simulink model "speed_control"  (R2024b)
settings: Solver=VariableStepAuto  StartTime=0.0  StopTime=10.0  RelTol=1e-3
values from neighbouring files (symbols this model uses):
  pmsm =     [foc.mat]    (also in inverter.mat; speed_control.mat; vbyf.mat)
  Ts = 2.5e-05    [foc.mat]    (also in inverter.mat; speed_control.mat; vbyf.mat)
libraries: mcbcontrollergainlib x2, mcbfoclib x1, mcbpositiondecoderlib x1, mcbplantlib x1, autolibpmsminterior x1, slpidlib x1
settings Model: Creator=realf  LastModifiedBy=realf

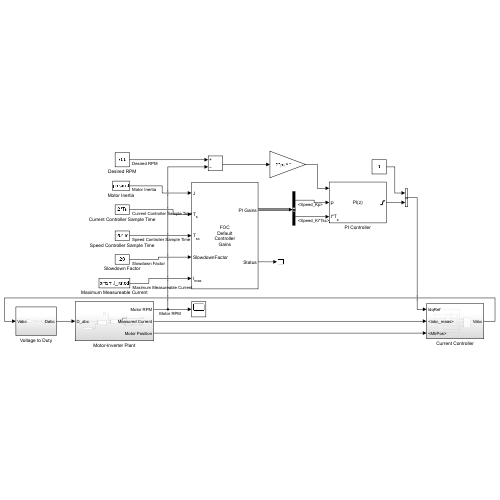
[thumbnail: Simulink's stored preview of the top-level diagram]
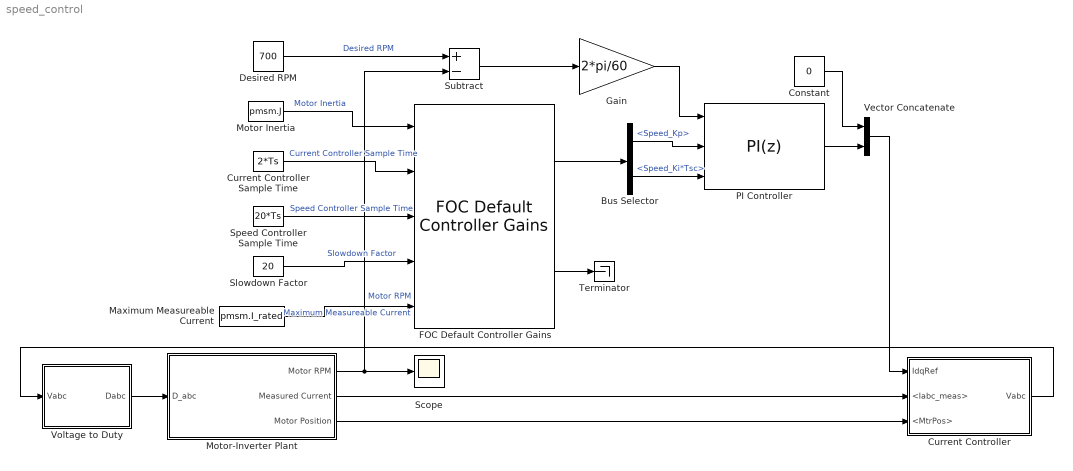
== system speed_control ==
  Bus Selector : BusSelector  OutputSignals=Speed_Kp,Speed_Ki*Tsc
  Constant : Constant  Value=0
  Current Controller : Subsystem
  Current Controller Sample Time : Constant  Value=2*Ts
  Desired RPM : Constant  Value=700
  FOC Default Controller Gains : mcbcontrollergainlib/FOC Default Controller Gains  motorSelection=PMSM  unitType=SI Unit  outCurrentControlGain=off  outFWCGain=off  outSpeedControlGain=on  externalDelay=off  currentSensorDelay=50e-6  speedSensorDelay=50e-6  speedFilterDelay=0.02
      settings: LibrarySourceBlock=mcblib/Controls/Controllers/FOC Default Controller Gains
  Gain : Gain  Gain=2*pi/60
  Maximum Measureable Current : Constant  Value=pmsm.I_rated
  Motor Inertia : Constant  Value=pmsm.J
  Motor-Inverter Plant : Subsystem
  PI Controller : slpidlib/PID Controller  Controller=PI  Form=Parallel  TimeDomain=Discrete-time  UseExternalTs=off  SampleTime=-1  IntegratorMethod=Forward Euler  FilterMethod=Forward Euler  ControllerParametersSource=external  P=1  I=1  UseKiTs=on  D=0  UseExternalDerivativeSource=off  N=100  UseFilter=on  TunerSelectOption=Transfer Function Based (PID Tuner App)  InitialConditionSource=internal  InitialConditionForIntegrator=0  InitialConditionForFilter=0  DifferentiatorICPrevScaledInput=0  ExternalReset=none  TrackingMode=off  Kt=1  LimitOutput=on  SatLimitsSource=internal  UpperSaturationLimit=pmsm.I_rated  LowerSaturationLimit=-pmsm.I_rated  LinearizeAsGain=on  AntiWindupMode=clamping  Kb=1  LimitIntegrator=on  UpperIntegratorSaturationLimit=pmsm.I_rated  LowerIntegratorSaturationLimit=-pmsm.I_rated  RndMeth=Simplest  POutMin=[]  POutMax=[]  IOutMin=[]  IOutMax=[]  DOutMin=[]  DOutMax=[]  NOutMin=[]  NOutMax=[]  SumOutMin=[]  SumOutMax=[]  SaturationOutDataTypeStr=Inherit: Inherit via back propagation  SaturationOutMin=[]  SaturationOutMax=[]  PParamMin=[]  PParamMax=[]  IParamMin=[]  IParamMax=[]  DParamMin=[]  DParamMax=[]  NParamMin=[]  NParamMax=[]  KbParamMin=[]  KbParamMax=[]  KtParamMin=[]  KtParamMax=[]  KbOutMin=[]  KbOutMax=[]  KtOutMin=[]  KtOutMax=[]  IntegratorOutMin=[]  IntegratorOutMax=[]  FilterOutMin=[]  FilterOutMax=[]  SumI1OutMin=[]  SumI1OutMax=[]  SumI2OutMin=[]  SumI2OutMax=[]  SumI3OutMin=[]  SumI3OutMax=[]  SumI4OutMin=[]  SumI4OutMax=[]  SumDOutMin=[]  SumDOutMax=[]  DifferentiatorOutMin=[]  DifferentiatorOutMax=[]  FilterDiffOutCoefMin=[]  FilterDiffOutCoefMax=[]  ReciprocalOutMin=[]  ReciprocalOutMax=[]  SumDenOutMin=[]  SumDenOutMax=[]  SumNumOutMin=[]  SumNumOutMax=[]  DivideOutMin=[]  DivideOutMax=[]  UdiffTsProdOutMin=[]  UdiffTsProdOutMax=[]  NTsProdOutMin=[]  NTsProdOutMax=[]  UintegralTsProdOutMin=[]  UintegralTsProdOutMax=[]  UngainTsProdOutMin=[]  UngainTsProdOutMax=[]  ClampingZeroOutDataTypeStr=Inherit: Inherit via back propagation  ClampingZeroOutMin=[]  ClampingZeroOutMax=[]  FilterDenConstantOutDataTypeStr=Inherit: Inherit via back propagation  FilterDenConstantOutMin=[]  FilterDenConstantOutMax=[]  PCopyOutDataTypeStr=Inherit: Inherit via back propagation  PCopyOutMin=[]  PCopyOutMax=[]  NCopyOutDataTypeStr=Inherit: Inherit via back propagation  NCopyOutMin=[]  NCopyOutMax=[]  IntegratorContinuousStateAttributes=''  IntegratorStateMustResolveToSignalObject=off  IntegratorRTWStateStorageClass=Auto  FilterContinuousStateAttributes=''  FilterStateMustResolveToSignalObject=off  FilterRTWStateStorageClass=Auto  ParallelPVariant=ExternalParameters  IdealPVariant=Disabled  IVariant=ExternalParameters  DVariant=Disabled  IntegratorVariant=Discrete  SatVariant=Enabled  AWVariant=DiscClampingParallel  PCopyVariant=Disabled  TRVariant=Disabled  FdbkBlocksVariant=Forward  IdealPFdbkVariant=Disabled  SatFdbkVariant=Disabled  DerivativeFilterVariant=Disabled  NVariant=Disabled  NCopyVariant=Disabled_SignalSpec  FilterICVariant=Disabled  IntegratorICVariant=InternalICs  ExternalResetVariant=Disabled  TRSumVariant=Passthrough  SumFdbkVariant=Disabled  SumVariant=Sum_PI  TsampFilterVariant=InternalTs  TsampNgainVariant=Passthrough  TsampIntegralVariant=Disabled_SignalSpec  ExternalSaturationOutDataTypeStr=Inherit: Same as second input  DerivativeSourceVariant=Disabled  PreIntVariant=InternalPreInt
      settings: LibrarySourceBlock=mcbhdllib/Controls/Controllers/PI Controller
  Scope : Scope
  Slowdown Factor : Constant  Value=20
  Speed Controller Sample Time : Constant  Value=20*Ts
  Subtract : Sum  Inputs=+-
  Terminator : Terminator
  Vector Concatenate : Concatenate
  Voltage to Duty : Subsystem
  wires:
  Voltage to Duty/1(Dabc) -> Motor-Inverter Plant/1(D_abc)
  Current Controller Sample Time/1 -> FOC Default Controller Gains/2  "Current Controller Sample Time"
  Constant/1 -> Vector Concatenate/1
  Desired RPM/1 -> Subtract/1  "Desired RPM"
  Motor-Inverter Plant/1(Motor RPM) -> Scope/1, Subtract/2  "Motor RPM"
  Maximum Measureable Current/1 -> FOC Default Controller Gains/5  "Maximum Measureable Current"
  Motor-Inverter Plant/2(Measured Current) -> Current Controller/2(<Iabc_meas>)
  Motor Inertia/1 -> FOC Default Controller Gains/1  "Motor Inertia"
  Slowdown Factor/1 -> FOC Default Controller Gains/4  "Slowdown Factor"
  PI Controller/1 -> Vector Concatenate/2
  Speed Controller Sample Time/1 -> FOC Default Controller Gains/3  "Speed Controller Sample Time"
  Motor-Inverter Plant/3(Motor Position) -> Current Controller/3(<MtrPos>)
  Subtract/1 -> Gain/1
  FOC Default Controller Gains/1 -> Bus Selector/1
  FOC Default Controller Gains/2 -> Terminator/1
  Gain/1 -> PI Controller/1
  Bus Selector/1 -> PI Controller/2  "<Speed_Kp>"
  Bus Selector/2 -> PI Controller/3  "<Speed_Ki*Tsc>"
  Vector Concatenate/1 -> Current Controller/1(IdqRef)
  Current Controller/1(Vabc) -> Voltage to Duty/1(Vabc)

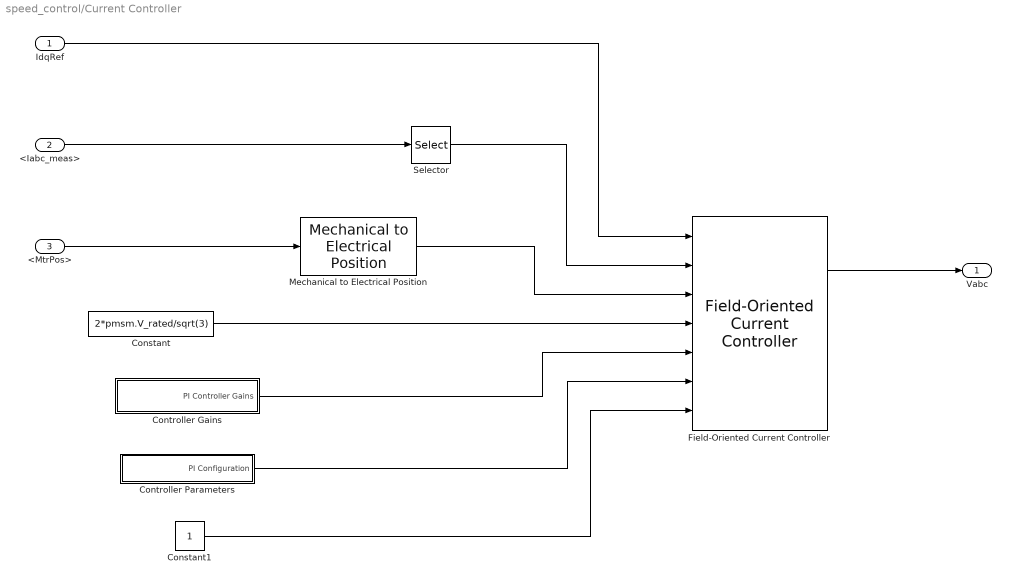
== system speed_control/Current Controller ==
  IdqRef : Inport
  <Iabc_meas> : Inport  Port=2
  <MtrPos> : Inport  Port=3
  Constant : Constant  Value=2*pmsm.V_rated/sqrt(3)
  Constant1 : Constant
  Controller Gains : Subsystem
  Controller Parameters : Subsystem
  Field-Oriented Current Controller : mcbfoclib/Field-Oriented Current Controller  AngleUnit=Radians  NumberOfLUTPoints=1024  AxisAlignment=D-axis  SaturationMethod=D-Q equivalence  PWMMethod=SVM: space vector modulation
  Mechanical to Electrical Position : mcbpositiondecoderlib/Mechanical to Electrical Position  PolePairsInputType=Specify via dialog  NrPP=pmsm.p  selectedRange=Radians  MechOfstInputType=Specify via dialog  mechOffsetIn=0  maxAngleIn=2*pi  InputDataType=single  VariantSelect=floating-point
  Selector : Selector  InputPortWidth=3  IndexOptions=Index vector (dialog)  Indices=[1 2]  OutputSizes=1
  Vabc : Outport
  wires:
  Field-Oriented Current Controller/1 -> Vabc/1
  <MtrPos>/1 -> Mechanical to Electrical Position/1
  IdqRef/1 -> Field-Oriented Current Controller/1
  <Iabc_meas>/1 -> Selector/1
  Controller Parameters/1(PI Configuration) -> Field-Oriented Current Controller/6
  Constant1/1 -> Field-Oriented Current Controller/7
  Selector/1 -> Field-Oriented Current Controller/2
  Constant/1 -> Field-Oriented Current Controller/4
  Controller Gains/1(PI Controller Gains) -> Field-Oriented Current Controller/5
  Mechanical to Electrical Position/1 -> Field-Oriented Current Controller/3

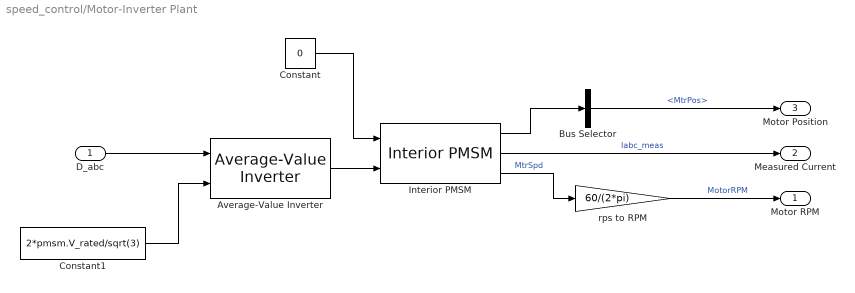
== system speed_control/Motor-Inverter Plant ==
  D_abc : Inport
  Average-Value Inverter : mcbplantlib/Average-Value Inverter
  Bus Selector : BusSelector  OutputSignals=MtrPos
  Constant : Constant  Value=0
  Constant1 : Constant  Value=2*pmsm.V_rated/sqrt(3)
  Interior PMSM : autolibpmsminterior/Interior PMSM  port_config=Torque  sim_type=Discrete  Ts=Ts  P=pmsm.p  Rs=pmsm.Rs  Ldq=[pmsm.Ld, pmsm.Lq]  KConstText=Permanent flux linkage constant (lambda_pm):  lambda_pm=pmsm.FluxPM  Ke=159.9771  mechanical=[pmsm.J, 0, 0]  idq0=[0 0]  theta_init=0  omega_init=0  KConst=pmsm.FluxPM  lambda_pm_calc=pmsm.FluxPM  Kt=0.07  RefBlkName='autolibpmsminterior/Interior PMSM'  aMode=5
  rps to RPM : Gain  Gain=60/(2*pi)
  Motor RPM : Outport
  Measured Current : Outport  Port=2
  Motor Position : Outport  Port=3
  wires:
  D_abc/1 -> Average-Value Inverter/1
  Interior PMSM/2 -> Measured Current/1  "Iabc_meas"
  Bus Selector/1 -> Motor Position/1  "<MtrPos>"
  Interior PMSM/1 -> Bus Selector/1
  Constant/1 -> Interior PMSM/1
  Constant1/1 -> Average-Value Inverter/2
  Average-Value Inverter/1 -> Interior PMSM/2
  rps to RPM/1 -> Motor RPM/1  "MotorRPM"
  Interior PMSM/3 -> rps to RPM/1  "MtrSpd"

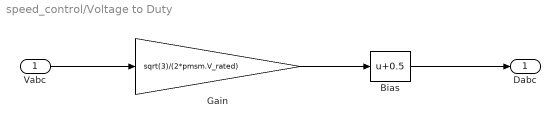
== system speed_control/Voltage to Duty ==
  Vabc : Inport
  Bias : Bias  Bias=0.5  SaturateOnIntegerOverflow=off
  Gain : Gain  Gain=sqrt(3)/(2*pmsm.V_rated)
  Dabc : Outport
  wires:
  Gain/1 -> Bias/1
  Vabc/1 -> Gain/1
  Bias/1 -> Dabc/1

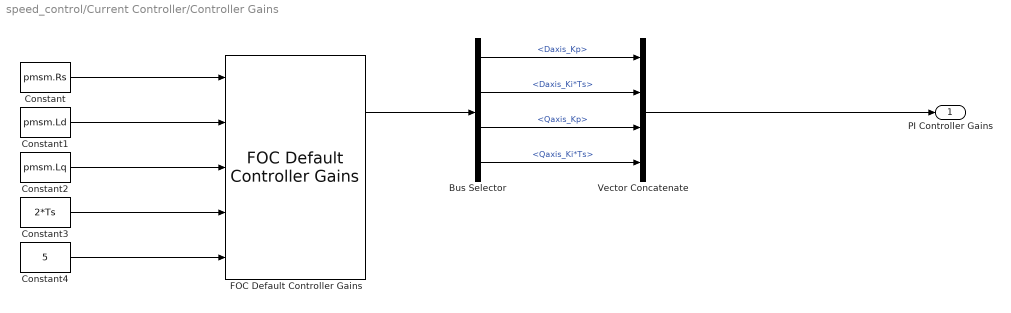
== system speed_control/Current Controller/Controller Gains ==
  Bus Selector : BusSelector  OutputSignals=Daxis_Kp,Daxis_Ki*Ts,Qaxis_Kp,Qaxis_Ki*Ts
  Constant : Constant  Value=pmsm.Rs
  Constant1 : Constant  Value=pmsm.Ld
  Constant2 : Constant  Value=pmsm.Lq
  Constant3 : Constant  Value=2*Ts
  Constant4 : Constant  Value=5
  FOC Default Controller Gains : mcbcontrollergainlib/FOC Default Controller Gains  motorSelection=PMSM  unitType=SI Unit  outCurrentControlGain=on  outFWCGain=off  outSpeedControlGain=off  externalDelay=off  currentSensorDelay=50e-6  speedSensorDelay=50e-6  speedFilterDelay=0.02
  Vector Concatenate : Concatenate  NumInputs=4
  PI Controller Gains : Outport
  wires:
  Vector Concatenate/1 -> PI Controller Gains/1
  Bus Selector/1 -> Vector Concatenate/1  "<Daxis_Kp>"
  Bus Selector/2 -> Vector Concatenate/2  "<Daxis_Ki*Ts>"
  Bus Selector/3 -> Vector Concatenate/3  "<Qaxis_Kp>"
  Bus Selector/4 -> Vector Concatenate/4  "<Qaxis_Ki*Ts>"
  FOC Default Controller Gains/1 -> Bus Selector/1
  Constant4/1 -> FOC Default Controller Gains/5
  Constant1/1 -> FOC Default Controller Gains/2
  Constant/1 -> FOC Default Controller Gains/1
  Constant2/1 -> FOC Default Controller Gains/3
  Constant3/1 -> FOC Default Controller Gains/4

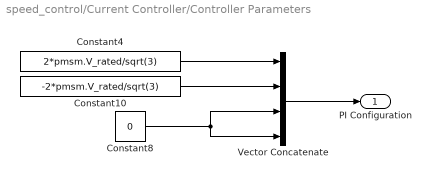
== system speed_control/Current Controller/Controller Parameters ==
  Constant10 : Constant  Value=-2*pmsm.V_rated/sqrt(3)
  Constant4 : Constant  Value=2*pmsm.V_rated/sqrt(3)  OutDataTypeStr=double
  Constant8 : Constant  Value=0
  Vector Concatenate : Concatenate  NumInputs=4
  PI Configuration : Outport
  wires:
  Constant4/1 -> Vector Concatenate/1
  Constant10/1 -> Vector Concatenate/2
  Constant8/1 -> Vector Concatenate/4, Vector Concatenate/3
  Vector Concatenate/1 -> PI Configuration/1
